simulink model "demux_vector_conv"  (Simulink 6.6)
settings: Solver=FixedStepDiscrete  StartTime=0.0  StopTime=10.0  FixedStep=1  RelTol=1e-3
settings Model: Creator=Administrator  LastModifiedBy=hnine
settings GRTTargetCC: TargetFcnLib=ansi_tfl_table_tmw.mat

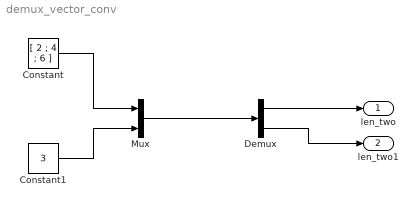
== system demux_vector_conv ==
  Constant : Constant  Value=[ 2 ; 4 ; 6 ]  VectorParams1D=off  OutDataTypeMode=single
  Constant1 : Constant  Value=3  VectorParams1D=off  OutDataTypeMode=single
  Demux : Demux  Outputs=[2,2]
  Mux : Mux  Inputs=[3,1]
  len_two : Outport  PortDimensions=[2]  DataType=single
  len_two1 : Outport  Port=2  PortDimensions=[2]  DataType=single
  wires:
  Constant/1 -> Mux/1
  Constant1/1 -> Mux/2
  Mux/1 -> Demux/1
  Demux/1 -> len_two/1
  Demux/2 -> len_two1/1
